simulink model "p1b1"  (R2023b)
settings: Solver=VariableStepAuto  StartTime=0.0  StopTime=2  RelTol=1e-3
settings Model: Creator=m96sz  LastModifiedBy=tanvi

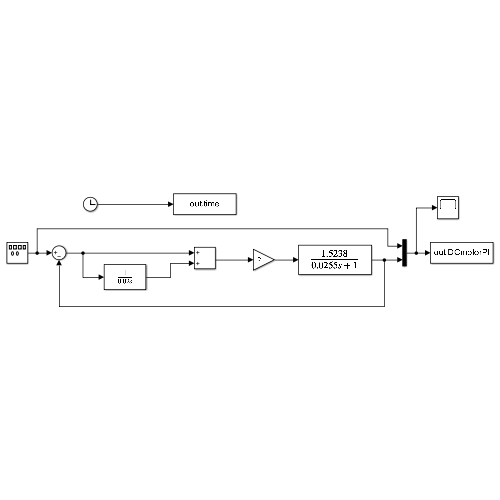
[thumbnail: Simulink's stored preview of the top-level diagram]
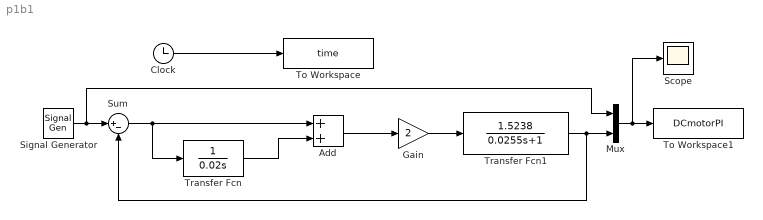
== system p1b1 ==
  Add : Sum
  Clock : Clock
  Gain : Gain  Gain=2
  Mux : Mux  Inputs=2
  Scope : Scope
  Signal Generator : SignalGenerator  WaveForm=square  Frequency=2
  Sum : Sum  Inputs=|+-
  To Workspace : ToWorkspace  VariableName=time  SampleTime=-1
  To Workspace1 : ToWorkspace  VariableName=DCmotorPI  SampleTime=-1
  Transfer Fcn : TransferFcn  Denominator=[0.02 0]
  Transfer Fcn1 : TransferFcn  Numerator=[1.5238]  Denominator=[0.0255 1]
  wires:
  Clock/1 -> To Workspace/1
  Signal Generator/1 -> Mux/1, Sum/1
  Sum/1 -> Transfer Fcn/1, Add/1
  Transfer Fcn/1 -> Add/2
  Add/1 -> Gain/1
  Gain/1 -> Transfer Fcn1/1
  Transfer Fcn1/1 -> Sum/2, Mux/2
  Mux/1 -> Scope/1, To Workspace1/1
